simulink model "BixlerTelemTest"  (R2018b)
settings: Solver=FixedStepAuto  StartTime=0.0  StopTime=inf  RelTol=1e-3  EnableMultiTasking=on
libraries: px4lib x2, px4Sensorslib x1
settings Model: SimulationMode=external  ExtModeTrigDuration=10  Creator=Robert  LastModifiedBy=Robert
settings SolverCC: PositivePriorityOrder=on
settings OptimizationCC: EnhancedBackFolding=on  PassReuseOutputArgsAs=Individual arguments  MaxStackSize=64  OptimizeBlockOrder=speed  DifferentSizesBufferReuse=on  OptimizationCustomize=off
settings DebuggingCC: ParameterTunabilityLossMsg=error
settings HardwareCC: ProdBitPerPointer=32  ProdBitPerSizeT=32  ProdBitPerPtrDiffT=32  ProdLargestAtomicInteger=Long  ProdLargestAtomicFloat=Double  ProdWordSize=32  ProdLongLongMode=on  ProdHWDeviceType=ARM Compatible->ARM Cortex
settings SFSimCC: MATLABDynamicMemAlloc=off
settings RTWCC: SystemTargetFile=ert.tlc  HardwareBoard=PX4 Pixhawk 1  TLCOptions="-aInlineSetEventsForThisBaseRateFcn=TLC_FALSE -aSuppressMultiTaskScheduler=TLC_FALSE  -aRateBasedStepFcn=0"  TemplateMakefile=ert_default_tmf  GenerateReport=on  Toolchain=GNU Tools for PX4 Autopilots  IncludeHyperlinkInReport=on  LaunchReport=on  TargetLang=C++  GenerateTraceInfo=on  GenerateTraceReport=on  GenerateTraceReportSl=on  GenerateTraceReportSf=on  GenerateTraceReportEml=on
settings CodeAppCC: ForceParamTrailComments=on  IgnoreCustomStorageClasses=off  OperatorAnnotations=on  SimulinkDataObjDesc=on  SFDataObjDesc=on  InsertBlockDesc=on
settings ERTTargetCC: ExtMode=on  ExtModeMexArgs='127.0.0.1' 1 17725

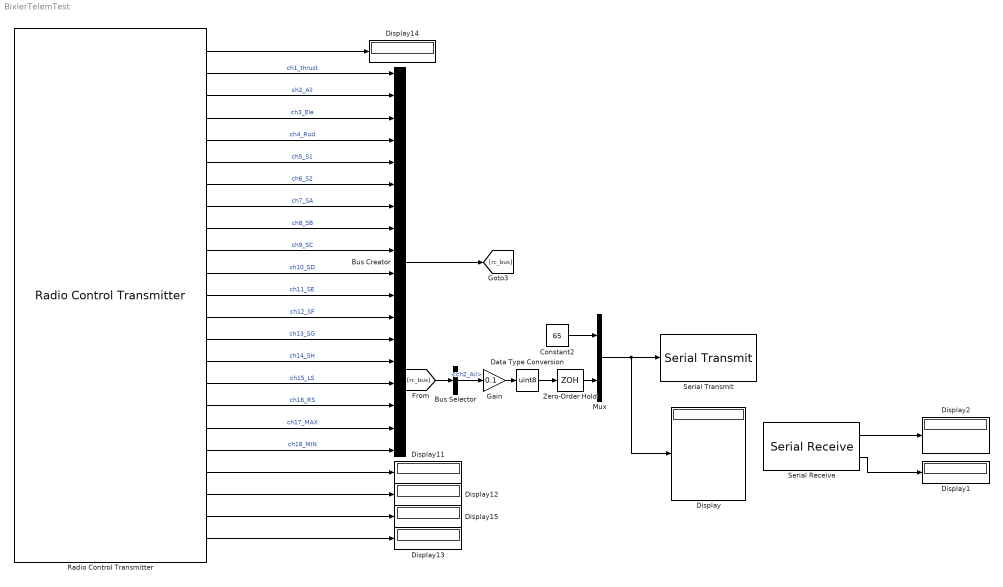
== system BixlerTelemTest ==
  Bus Creator : BusCreator  Inputs=18
  Bus Selector : BusSelector  OutputSignals=ch2_Ail
  Constant2 : Constant  Value=65  OutDataTypeStr=uint8  SampleTime=0.1
  Data Type Conversion : DataTypeConversion  OutDataTypeStr=uint8
  Display{,1..2,11..15} (8 alike) : Display
  Gain : Gain  Gain=0.1
  Mux : Mux  Inputs=2
  Radio Control Transmitter : px4Sensorslib/Radio Control Transmitter  channel1=on  channel2=on  channel3=on  channel4=on  channel5=on  channel6=on  channel7=on  channel8=on  channel9=on  channel10=on  channel11=on  channel12=on  channel13=on  channel14=on  channel15=on  channel16=on  channel17=on  channel18=on  channel_count=on  rssi=on  rc_input_source=on  timestamp_last_signal=on  time_stamp=off  sampleTime=1/250  BlockingMode=off  BlockTimeout=5
      settings: SourceProductName=Embedded Coder Support Package for PX4 Autopilots
  Serial Receive : px4lib/Serial Receive  SCIModule=/dev/ttyS2  DataType=uint8  DataLength=2  OutputStatus=on  SampleTime=0.1  BlockingMode=off  PartialData=off  Timeout=5
      settings: SourceProductName=Embedded Coder Support Package for PX4 Autopilots
  Serial Transmit : px4lib/Serial Transmit  SCIModule=/dev/ttyS2
      settings: SourceProductName=Embedded Coder Support Package for PX4 Autopilots
  Zero-Order Hold : ZeroOrderHold  SampleTime=0.1
  wires:
  Radio Control Transmitter/8 -> Bus Creator/7  "ch7_SA"
  Radio Control Transmitter/7 -> Bus Creator/6  "ch6_S2"
  Radio Control Transmitter/6 -> Bus Creator/5  "ch5_S1"
  Radio Control Transmitter/2 -> Bus Creator/1  "ch1_thrust"
  Radio Control Transmitter/3 -> Bus Creator/2  "ch2_Ail"
  Radio Control Transmitter/4 -> Bus Creator/3  "ch3_Ele"
  Radio Control Transmitter/5 -> Bus Creator/4  "ch4_Rud"
  Radio Control Transmitter/9 -> Bus Creator/8  "ch8_SB"
  Radio Control Transmitter/20 -> Display11/1
  Radio Control Transmitter/21 -> Display12/1
  Radio Control Transmitter/23 -> Display13/1
  Radio Control Transmitter/1 -> Display14/1
  Radio Control Transmitter/22 -> Display15/1
  Bus Creator/1 -> [rc_bus]
  Radio Control Transmitter/10 -> Bus Creator/9  "ch9_SC"
  Radio Control Transmitter/11 -> Bus Creator/10  "ch10_SD"
  Radio Control Transmitter/12 -> Bus Creator/11  "ch11_SE"
  Radio Control Transmitter/13 -> Bus Creator/12  "ch12_SF"
  Radio Control Transmitter/14 -> Bus Creator/13  "ch13_SG"
  Radio Control Transmitter/15 -> Bus Creator/14  "ch14_SH"
  Radio Control Transmitter/16 -> Bus Creator/15  "ch15_LS"
  Radio Control Transmitter/17 -> Bus Creator/16  "ch16_RS"
  Radio Control Transmitter/18 -> Bus Creator/17  "ch17_MAX"
  Radio Control Transmitter/19 -> Bus Creator/18  "ch18_MIN"
  Constant2/1 -> Mux/1
  [rc_bus] -> Bus Selector/1
  Bus Selector/1 -> Gain/1  "<ch2_Ail>"
  Gain/1 -> Data Type Conversion/1
  Data Type Conversion/1 -> Zero-Order Hold/1
  Mux/1 -> Display/1, Serial Transmit/1
  Serial Receive/2 -> Display1/1
  Serial Receive/1 -> Display2/1
  Zero-Order Hold/1 -> Mux/2
